simulink library "pixhawk_slib_rfly"  (R2022b)
settings: Solver=ode45  StartTime=0.0  StopTime=10.0  RelTol=1e-3
libraries: pixhawk_slib_uORB_RW x42, $bdroot x7
(part 3 of 3)

== matlab function pixhawk_slib_rfly/OffboardAdvCtrlAPI/CmdGenerator ==
  data: isEnCtrl input; cmd output; params1 output; params2 output; params3 output; isSendCmd output; t input; isSendOff output; isAutoArm input; isAutoBlock input; isSendBlock output; isAutoLoiter input
function [cmd,params1,params2,params3,isSendCmd,isSendOff,isSendBlock] = fcn(isEnCtrl,t,isAutoArm,isAutoBlock,isAutoLoiter)


persistent lastT;
persistent flag;
persistent lastEnCtrl;

isSendBlock=false;

if isempty(lastT)
    lastT=0;
end

if isempty(flag)
    flag=0;
end



if isempty(lastEnCtrl)
    lastEnCtrl=false;
    if isAutoBlock
        isSendBlock=true;
    end
end

isSendCmd=0;
isSendOff=0;

cmd=uint32(0);
params1=single(NaN);
params2=single(NaN);
params3=single(NaN);



if lastEnCtrl~= isEnCtrl% 不相等
    lastEnCtrl = isEnCtrl;
    
    if isAutoBlock
        isSendBlock=true;
    end
    
    
    if isEnCtrl % 使能Offboard
        if isAutoArm
            flag=1; % 进入等待Offboard模式切换指令            
        else
            flag=3; % 直接进入发送数据模式
        end

        
    else % 禁用Offboard
        
        flag=0;
        if isAutoLoiter % 如果启用自动悬停，就进入悬停模式
            isSendCmd=1; % 发送命令
            cmd=uint32(176); %MAV_CMD_DO_SET_MODE
            params1=single(1); % Mode
            params2=single(4); % Custom Mode: PX4_CUSTOM_MAIN_MODE_AUTO
            params3=single(3); % Custom Submode: PX4_CUSTOM_SUB_MODE_AUTO_LOITER
            % 切换到定点模式
        end

    end
    
    lastT=t;
end

if abs(flag-1)<0.01 && (t-lastT)>1.2  % 发送offboard数据2秒后，切换Offboard模式
    flag=2;
    isSendCmd=1; % 发送命令
    cmd=uint32(176); %MAV_CMD_DO_SET_MODE
    params1=single(1); % Mode
    params2=single(6); % Custom Mode: PX4_CUSTOM_MAIN_MODE_OFFBOARD
end


if abs(flag-2)<0.01 && (t-lastT)>2.2  % 切换Offboard1秒后，尝试发送解锁指令
    flag=3;
    isSendCmd=1; % 发送命令
    cmd=uint32(400); %MAV_CMD_COMPONENT_ARM_DISARM
    params1=single(1); %  Arm
    params2=single(0); %  No Force
end

% 只要在Offboard发送模式，就发送Offboard消息
if flag>0.5 && flag<3.5
    isSendOff=1; % 开始发送Offboard消息
end

== matlab function pixhawk_slib_rfly/OffboardAdvCtrlAPI/MATLAB Function ==
  data: u input; idxList input; y output
function y = fcn(u,idxList)
y=single(NaN(11,1));
uLen=length(u);
idxLen=length(idxList);

minLen=uLen;
if idxLen<uLen
    minLen=idxLen;
end

if minLen>0.5
    for i=1:minLen
        y(idxList(i))=u(i);
    end
end

== matlab function pixhawk_slib_rfly/OffboardAttCtrlAPI/CmdGenerator ==
  data: isEnCtrl input; cmd output; params1 output; params2 output; params3 output; isSendCmd output; t input; isSendOff output; isAutoArm input; isAutoBlock input; isSendBlock output; isAutoLoiter input
function [cmd,params1,params2,params3,isSendCmd,isSendOff,isSendBlock] = fcn(isEnCtrl,t,isAutoArm,isAutoBlock,isAutoLoiter)


persistent lastT;
persistent flag;
persistent lastEnCtrl;


isSendBlock=false;

if isempty(lastT)
    lastT=0;
end

if isempty(flag)
    flag=0;
end


if isempty(lastEnCtrl)
    lastEnCtrl=false;
    if isAutoBlock
        isSendBlock=true;
    end
end

isSendCmd=0;
isSendOff=0;

cmd=uint32(0);
params1=single(NaN);
params2=single(NaN);
params3=single(NaN);



if lastEnCtrl~= isEnCtrl% 不相等
    lastEnCtrl = isEnCtrl;
    
    if isAutoBlock
        isSendBlock=true;
    end
    
    
    if isEnCtrl % 使能Offboard
        if isAutoArm
            flag=1; % 进入等待Offboard模式切换指令            
        else
            flag=3; % 直接进入发送数据模式
        end
        
    else % 禁用Offboard
        
        flag=0;
        if isAutoLoiter % 如果启用自动悬停，就进入悬停模式
            isSendCmd=1; % 发送命令
            cmd=uint32(176); %MAV_CMD_DO_SET_MODE
            params1=single(1); % Mode
            params2=single(4); % Custom Mode: PX4_CUSTOM_MAIN_MODE_AUTO
            params3=single(3); % Custom Submode: PX4_CUSTOM_SUB_MODE_AUTO_LOITER
            % 切换到定点模式
        end

    end
    
    lastT=t;
end

if abs(flag-1)<0.01 && (t-lastT)>1.2  % 发送offboard数据2秒后，切换Offboard模式
    flag=2;
    isSendCmd=1; % 发送命令
    cmd=uint32(176); %MAV_CMD_DO_SET_MODE
    params1=single(1); % Mode
    params2=single(6); % Custom Mode: PX4_CUSTOM_MAIN_MODE_OFFBOARD
end


if abs(flag-2)<0.01 && (t-lastT)>2.2  % 切换Offboard1秒后，尝试发送解锁指令
    flag=3;
    isSendCmd=1; % 发送命令
    cmd=uint32(400); %MAV_CMD_COMPONENT_ARM_DISARM
    params1=single(1); %  Arm
    params2=single(0); %  No Force
end

% 只要在Offboard发送模式，就发送Offboard消息
if flag>0.5 && flag<3.5
    isSendOff=1; % 开始发送Offboard消息
end
